simulink model "IO301interruptsynch"  (R2013a)
settings: Solver=FixedStepDiscrete  StartTime=0.0  StopTime=inf  RelTol=1e-3
PreLoadFcn:
  | fpga_freq = 33e6;
  | Tpwm = 100e-6;
libraries: speedgoatlib_IO301 x3, xpclib x1
settings Model: BufferReuse=off  Creator=dkuratli  LastModifiedBy=lab3
settings SolverCC: EnableConcurrentExecution=on
settings OptimizationCC: BlockReduction=off  OptimizeBlockIOStorage=off  BufferReuse=off  ExpressionFolding=off  LocalBlockOutputs=off
settings DebuggingCC: UnderspecifiedInitializationDetection=Simplified  StateNameClashWarn=none
settings HardwareCC: ProdIntDivRoundTo=Zero  ProdEndianess=LittleEndian  ProdHWDeviceType=Generic->32-bit x86 compatible
settings RTWCC: SystemTargetFile=xpctarget.tlc  TemplateMakefile=xpc_default_tmf  Description=Simulink Real-Time  RTWVerbose=off  ProcessScript=xpctarget_make_rtw_hook  RTWCompilerOptimization=On
settings xpcTargetCC: TargetFcnLib=ansi_tfl_table_tmw.mat  CodeReplacementLibrary=XPC_BLAS  ParMdlRefBuildCompliant=on  ConcurrentExecutionCompliant=on  CombineSignalStateStructs=off  MATLABClassNameForMDSCustomization=xpcAperiodicCustomization  GRTInterface=on  GenerateAllocFcn=off  xPCTaskExecutionProfile=off  xPCRL32EventNumber=5000  RL32IRQSourceModifier=Auto (PCI only)  xPCLoadParamSetFile=off  xPCConcurrentTasks=off  xPCEnableSFAnimation=off

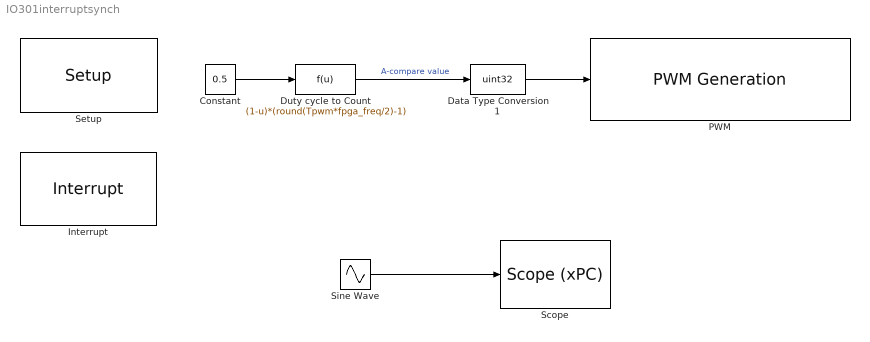
== system IO301interruptsynch ==
  Constant : Constant  Value=0.5  SampleTime=Tpwm
  Data Type Conversion1 : DataTypeConversion  OutDataTypeStr=uint32
  Duty cycle to Count : Fcn  Expr=(1-u)*(round(Tpwm*fpga_freq/2)-1)
  Interrupt : speedgoatlib_IO301/Interrupt/Interrupt  id=1  debounce=0  delay=0  polarity=0  pciSlot=-1  ts=-1
  PWM : speedgoatlib_IO301/PWM Generation/PWM Generation  channel=[1]  group=Module setup  id=1  ts=-1  pciSlot=-1  initStart=[1]  toggleAStart=[0]  toggleAStop=[0]  toggleBStart=[1]  toggleBStop=[0]  showStart=off  showAStart=off  showAStop=off  showBStart=off  showBStop=off  initA=[1]  initB=[1]  initC=[round(fpga_freq*Tpwm/2)-1]  showA=on  showB=off  showC=off  initActionA=[0,0,2,1]'  initActionB=[0,0,2,1]'  showActionA=off  showActionB=off  triggerSource=[1]  triggerPulseLength=32  protection=[0]
  "Scope " : xpclib/Misc./Scope (xPC)   scopeno=1  scopetype=Target  autostart=on  viewmode=Graphical redraw  formatstr='%15.6f'  grid=on  ylimits=[0,0]  nosamples=250  noprepostsamples=0  interleave=1  triggermode=FreeRun  triggersignal=1  trigsignalfromport=off  triggerlevel=0.0  triggerslope=Either  triggerscope=1  triggersample=0  filename=data.dat  mode=Lazy  writesize=512  autorestart=off  dynamicfilemode=off  maxwritefilesize=512*1024^2
  Setup : speedgoatlib_IO301/Setup/Setup  group=Module setup  id=1  fpga1=speedgoat_IO301_default  pciSlot=-1  lowerDirection=[1, 1, 1, 1, 1, 0, 0, 0, 0, 0, 0, 0, 1, 1, 1, 1]  lowerReset=[1]  lowerValue=[0]  upperDirection=[1, 1, 1, 1, 1, 1, 1, 1, 0, 0, 0, 0, 0, 0, 0, 0]  upperReset=[1]  upperValue=[0]
  Sine Wave : Sin  Amplitude=[1, 2, 3]  Frequency=2*pi*100  SampleTime=Tpwm
  wires:
  Duty cycle to Count/1 -> Data Type Conversion1/1  "A-compare value"
  Data Type Conversion1/1 -> PWM/1
  Constant/1 -> Duty cycle to Count/1
  Sine Wave/1 -> "Scope "/1
